simulink model "figure7"  (R2015b)
settings: Solver=FixedStepAuto  StartTime=0.0  StopTime=10  RelTol=1e-3
values from neighbouring files (symbols this model uses):
  bHI = 35    [Initiation.m]
  bWall = 0    [Initiation.m]    (also in VirtualEnvironment.m = block.DialogPrm(2).Data; Virtual_Environment.m = block.DialogPrm(2).Data)
  kWall = 90000    [Initiation.m]    (also in VirtualEnvironment.m = block.DialogPrm(1).Data; Virtual_Environment.m = block.DialogPrm(1).Data)
  m = 1    [Initiation.m]
  nWall = 1    [Initiation.m]    (also in VirtualEnvironment.m = block.DialogPrm(3).Data; Virtual_Environment.m = block.DialogPrm(3).Data)
  tsampling = 0.001    [Initiation.m]    (also in VirtualEnvironment.m = block.DialogPrm(6).Data; Virtual_Environment.m = block.DialogPrm(6).Data)
  x0 = 0.14    [Initiation.m]    (also in PC.m = []; Wall.m = []; devision.m = []; sgn.m = [])
  x_dot0 = 0    [Initiation.m]
  xWall = 0.085    [Initiation.m]
libraries: simulink x4
settings Model: Creator=TOSHIBA  LastModifiedBy=TOSHIBA

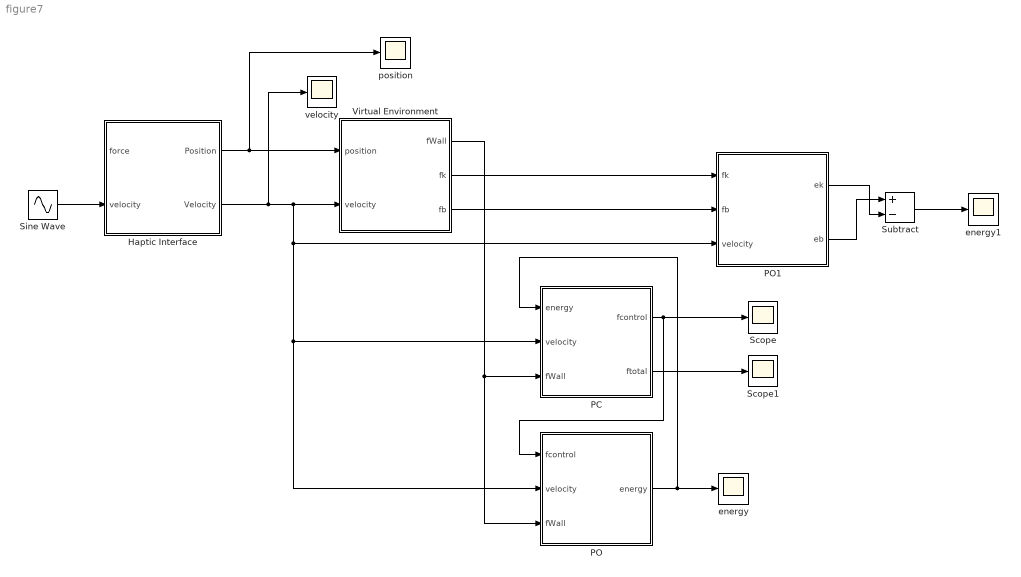
== system figure7 ==
  Haptic Interface : Subsystem
  PC : Subsystem
  PO : Subsystem
  PO1 : Subsystem
  Scope : Scope
  Scope1 : Scope
  Sine Wave : Sin  Frequency=pi  SampleTime=0
  Subtract : Sum  Inputs=+-
  Virtual Environment : Subsystem
  energy : Scope
  energy1 : Scope
  position : Scope
  velocity : Scope
  wires:
  Haptic Interface/1(Position) -> position/1, Virtual Environment/1(position)
  Haptic Interface/2(Velocity) -> PO/2(velocity), PC/2(velocity), PO1/3(velocity), Virtual Environment/2(velocity), velocity/1
  PC/2(ftotal) -> Scope1/1
  PO/1(energy) -> energy/1, PC/1(energy)
  PC/1(fcontrol) -> Scope/1, PO/1(fcontrol)
  Sine Wave/1 -> Haptic Interface/2(velocity)
  Virtual Environment/1(fWall) -> PO/3(fWall), PC/3(fWall)
  Virtual Environment/2(fk) -> PO1/1(fk)
  Virtual Environment/3(fb) -> PO1/2(fb)
  PO1/2(eb) -> Subtract/1
  PO1/1(ek) -> Subtract/2
  Subtract/1 -> energy1/1

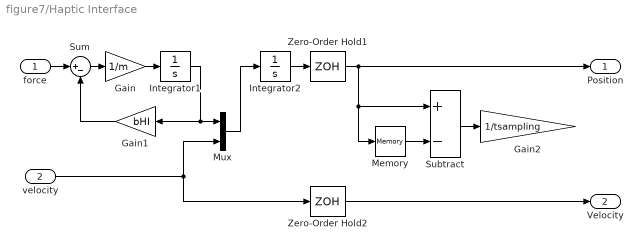
== system figure7/Haptic Interface ==
  force : Inport
  velocity : Inport  Port=2
  Gain : Gain  Gain=1/m
  Gain1 : Gain  Gain=bHI
  Gain2 : Gain  Gain=1/tsampling
  Integrator1 : Integrator  InitialCondition=x_dot0
  Integrator2 : Integrator  InitialCondition=x0
  Memory : Memory  X0=x0
  Mux : Mux  Inputs=2
  Subtract : Sum  Inputs=+-
  Sum : Sum  Inputs=|+-
  Zero-Order Hold1 : ZeroOrderHold  SampleTime=tsampling
  Zero-Order Hold2 : ZeroOrderHold  SampleTime=tsampling
  Position : Outport
  Velocity : Outport  Port=2
  wires:
  Subtract/1 -> Gain2/1
  Memory/1 -> Subtract/2
  Zero-Order Hold1/1 -> Position/1, Memory/1, Subtract/1
  Integrator2/1 -> Zero-Order Hold1/1
  Gain1/1 -> Sum/2
  Integrator1/1 -> Mux/1, Gain1/1
  Gain/1 -> Integrator1/1
  force/1 -> Sum/1
  Sum/1 -> Gain/1
  velocity/1 -> Zero-Order Hold2/1, Mux/2
  Mux/1 -> Integrator2/1
  Zero-Order Hold2/1 -> Velocity/1

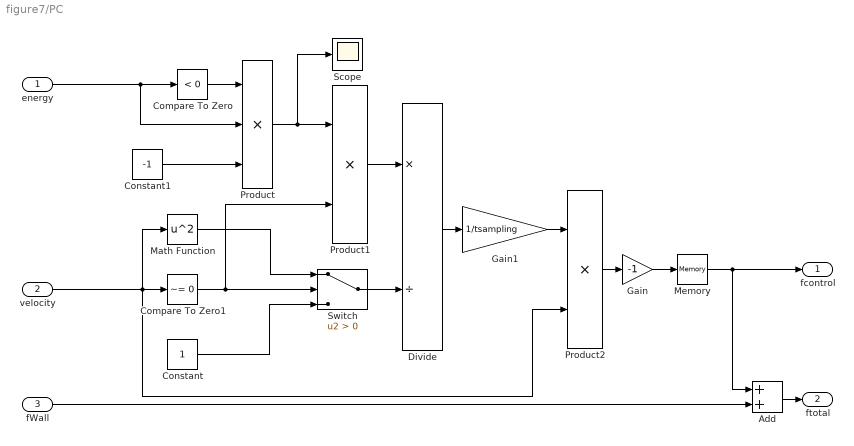
== system figure7/PC ==
  energy : Inport
  velocity : Inport  Port=2
  fWall : Inport  Port=3
  Add : Sum
  Compare To Zero : simulink/Logic and Bit Operations/Compare To Zero  relop=<  OutDataTypeStr=boolean
  Compare To Zero1 : simulink/Logic and Bit Operations/Compare To Zero  relop=~=  OutDataTypeStr=boolean
  Constant : Constant
  Constant1 : Constant  Value=-1
  Divide : Product  Inputs=*/
  Gain : Gain  Gain=-1
  Gain1 : Gain  Gain=1/tsampling
  Math Function : Math  Operator=square  SaturateOnIntegerOverflow=on
  Memory : Memory
  Product : Product  Inputs=3
  Product1 : Product
  Product2 : Product
  Scope : Scope
  Switch : Switch  Criteria=u2 > Threshold
  fcontrol : Outport
  ftotal : Outport  Port=2
  wires:
  velocity/1 -> Math Function/1, Product2/2, Compare To Zero1/1
  Compare To Zero/1 -> Product/1
  Compare To Zero1/1 -> Product1/2, Switch/2
  Constant/1 -> Switch/3
  Math Function/1 -> Switch/1
  Gain1/1 -> Product2/1
  Divide/1 -> Gain1/1
  Product1/1 -> Divide/1
  Product2/1 -> Gain/1
  Switch/1 -> Divide/2
  Add/1 -> ftotal/1
  fWall/1 -> Add/2
  Product/1 -> Scope/1, Product1/1
  energy/1 -> Product/2, Compare To Zero/1
  Constant1/1 -> Product/3
  Gain/1 -> Memory/1
  Memory/1 -> Add/1, fcontrol/1

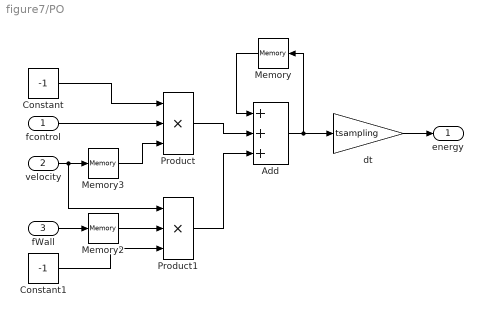
== system figure7/PO ==
  fcontrol : Inport
  velocity : Inport  Port=2
  fWall : Inport  Port=3
  Add : Sum  Inputs=+++
  Constant : Constant  Value=-1
  Constant1 : Constant  Value=-1
  Memory : Memory
  Memory2 : Memory
  Memory3 : Memory
  Product : Product  Inputs=3
  Product1 : Product  Inputs=3
  dt : Gain  Gain=tsampling
  energy : Outport
  wires:
  Add/1 -> dt/1, Memory/1
  Memory/1 -> Add/1
  Product/1 -> Add/2
  dt/1 -> energy/1
  Constant/1 -> Product/1
  fWall/1 -> Memory2/1
  Constant1/1 -> Product1/3
  Product1/1 -> Add/3
  Memory2/1 -> Product1/2
  velocity/1 -> Memory3/1, Product1/1
  fcontrol/1 -> Product/2
  Memory3/1 -> Product/3

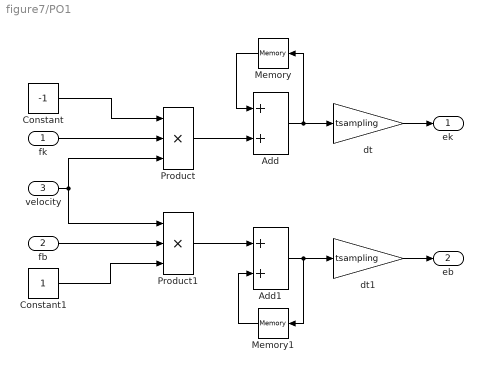
== system figure7/PO1 ==
  fk : Inport
  fb : Inport  Port=2
  velocity : Inport  Port=3
  Add : Sum
  Add1 : Sum
  Constant : Constant  Value=-1
  Constant1 : Constant
  Memory : Memory
  Memory1 : Memory
  Product : Product  Inputs=3
  Product1 : Product  Inputs=3
  dt : Gain  Gain=tsampling
  dt1 : Gain  Gain=tsampling
  ek : Outport
  eb : Outport  Port=2
  wires:
  Constant1/1 -> Product1/3
  fb/1 -> Product1/2
  velocity/1 -> Product/3, Product1/1
  fk/1 -> Product/2
  Constant/1 -> Product/1
  Product/1 -> Add/2
  Memory/1 -> Add/1
  Add/1 -> dt/1, Memory/1
  Add1/1 -> Memory1/1, dt1/1
  Memory1/1 -> Add1/2
  Product1/1 -> Add1/1
  dt/1 -> ek/1
  dt1/1 -> eb/1

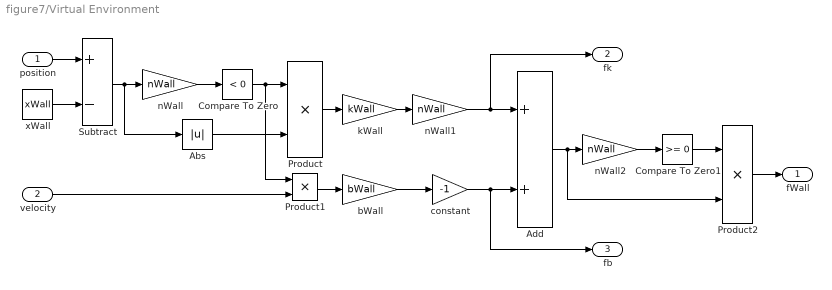
== system figure7/Virtual Environment ==
  position : Inport
  velocity : Inport  Port=2
  Abs : Abs
  Add : Sum
  Compare To Zero : simulink/Logic and Bit Operations/Compare To Zero  relop=<  OutDataTypeStr=boolean
  Compare To Zero1 : simulink/Logic and Bit Operations/Compare To Zero  relop=>=  OutDataTypeStr=boolean
  Product : Product
  Product1 : Product
  Product2 : Product
  Subtract : Sum  Inputs=+-
  bWall : Gain  Gain=bWall
  constant : Gain  Gain=-1
  kWall : Gain  Gain=kWall
  nWall : Gain  Gain=nWall
  nWall1 : Gain  Gain=nWall
  nWall2 : Gain  Gain=nWall
  xWall : Constant  Value=xWall
  fWall : Outport
  fk : Outport  Port=2
  fb : Outport  Port=3
  wires:
  xWall/1 -> Subtract/2
  position/1 -> Subtract/1
  Subtract/1 -> Abs/1, nWall/1
  nWall/1 -> Compare To Zero/1
  Compare To Zero/1 -> Product1/1, Product/1
  Abs/1 -> Product/2
  Product/1 -> kWall/1
  kWall/1 -> nWall1/1
  bWall/1 -> constant/1
  constant/1 -> fb/1, Add/2
  nWall1/1 -> fk/1, Add/1
  Product1/1 -> bWall/1
  velocity/1 -> Product1/2
  Add/1 -> Product2/2, nWall2/1
  nWall2/1 -> Compare To Zero1/1
  Compare To Zero1/1 -> Product2/1
  Product2/1 -> fWall/1
